simulink model "AdaptiveSIL"  (R2024a)
settings: Solver=VariableStepAuto  StartTime=0.0  StopTime=10  RelTol=1e-3
values from neighbouring files (symbols this model uses):
  am = 1/(Rlnom*C)    (= 53.1914893617)    [params.m]
  bm = 1    [params.m]
  C = 470e-6    (= 0.00047)    [params.m]
  k1 = 5000000    [params.m]
  k2 = 400000    [params.m]
  k3 = 700000    [params.m]
  kappa = 320    [params.m]
  L = 0.5e-3    (= 0.0005)    [params.m]
  omega = 100*pi    (= 314.159265359)    [params.m]
  Qas = bm    (= 1)    [params.m]
  R = 0.1    [params.m]
  Rlnom = 40    [params.m]
  Thetaas = 0    [params.m]
  vod = 200    [params.m]
libraries: eeTransforms x2, pspsim x1, spsSVPWMGenerator2LevelLib x1, spspowerguiLib x1
settings Model: Creator=CIO  LastModifiedBy=rodol
settings DebuggingCC: UnconnectedInputMsg=warning  UnconnectedOutputMsg=warning  UnconnectedLineMsg=warning
settings ModelReferenceCC: EnableRefExpFcnMdlSchedulingChecks=on
settings RTWCC: GPUComputeCapability=3.5  DLArmComputeVersion=19.05

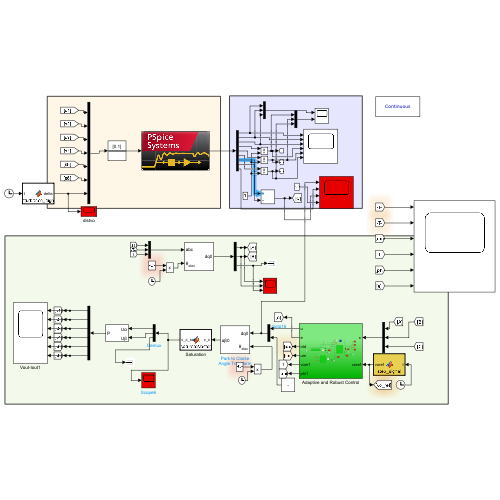
[thumbnail: Simulink's stored preview of the top-level diagram]
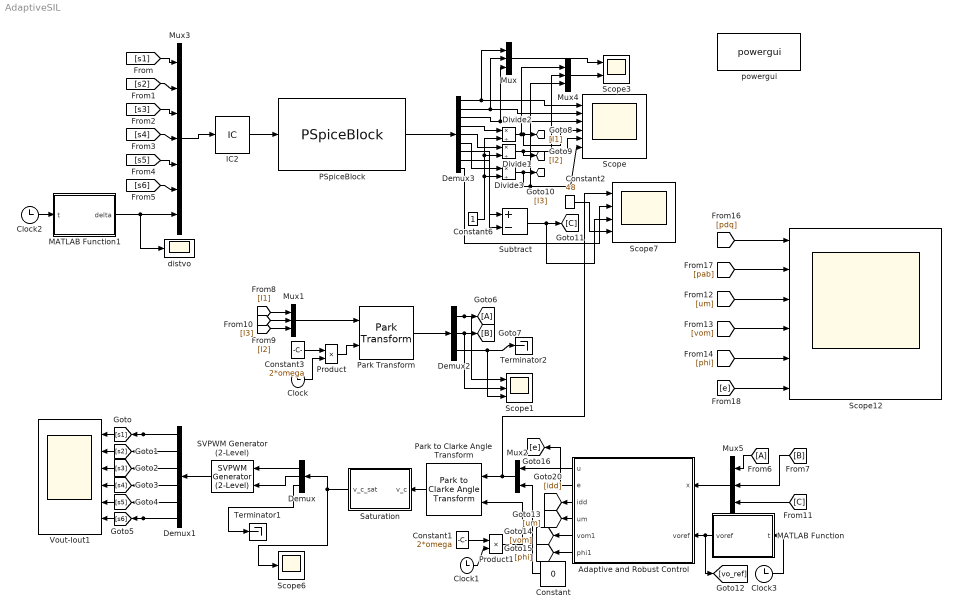
== system AdaptiveSIL ==
  Adaptive and Robust Control : Subsystem
  Clock{,1..3} (4 alike) : Clock
  Constant : Constant  Value=0
  Constant1 : Constant  Value=2*omega
  Constant2 : Constant  Value=48
  Constant3 : Constant  Value=2*omega
  Constant6 : Constant
  Demux : Demux  Outputs=3
  Demux1 : Demux  Outputs=6
  Demux2 : Demux  Outputs=3
  Demux3 : Demux  Outputs=9
  Divide1 : Product  Inputs=*/
  Divide2 : Product  Inputs=*/
  Divide3 : Product  Inputs=*/
  From6 : From
  Goto6 : Goto
  IC2 : InitialCondition  Value=0.1
  MATLAB Function : MATLAB Function  TreatAsAtomicUnit=on
  MATLAB Function1 : MATLAB Function  TreatAsAtomicUnit=on
  Mux{,1,4..5} (4 alike) : Mux  Inputs=3
  Mux2 : Mux  Inputs=2
  Mux3 : Mux  Inputs=7
  PSpiceBlock : pspsim/PSpiceBlock  SFunctionModules=''
      settings: SourceProductName=PSpice Block
  Park Transform : eeTransforms/Park Transform  AxisAlignment=D-axis  PowerInvariant=off
  Park to Clarke Angle Transform : eeTransforms/Park to Clarke Angle Transform  AxisAlignment=D-axis
  Product : Product
  Product1 : Product
  SVPWM Generator (2-Level) : spsSVPWMGenerator2LevelLib/SVPWM Generator (2-Level)  InputType=alpha-beta components  SwitchingPattern=Pattern #1  Fc=10000  ParUref=[0.8 -30 50]  Ts=0
  Saturation : MATLAB Function  TreatAsAtomicUnit=on
  Scope : Scope  NumInputPorts=6
  Scope1 : Scope  NumInputPorts=3
  Scope12 : Scope  NumInputPorts=6
  Scope3 : Scope  NumInputPorts=2
  Scope6 : Scope
  Scope7 : Scope  NumInputPorts=4
  Subtract : Sum  Inputs=+-
  Terminator1 : Terminator
  Terminator2 : Terminator
  Vout-Iout1 : Scope  NumInputPorts=6
  distvo : Scope
  powergui : spspowerguiLib/powergui  Priority=1  SimulationMode=Continuous  SampleTime=2e-6  frequency=60  Iterations=50  frequencyindice=60  Pbase=100e6  ErrMax=1e-4  UnitsV=kV  UnitsW=MW  buscounter=0  FunctionMessages=off  echomessages=off  EnableUseOfTLC=off  CurrentSourceSwitches=off  DisableSnubberDevices=off  DisableRonSwitches=off  DisableVfSwitches=off  DisplayEquations=off  AutomaticDiscreteSolvers=off  SolverType=Tustin/Backward Euler (TBE)  Interpol=off  ExternalGateDelay=off  methode=off  Ts=0  x0status=blocks  SPID=off  SwTol=0  HookPort=off  NonlinearTolerance=0  nMaxIteration=15  ContinueOnMaxIteration=off  RestoreLinks=warning  ResistiveCurrentMeasurement=off  Frange=[0:2:500]  Ylog=off  Xlog=on  ShowGrid=off  save=off  variable=ZData  structure=0  ZoomFFT=on  StartTime=0.0  cycles=1  DisplayStyle=1  fundamental=60  FreqAxis=off  MaxFrequency=1000  frequencyindicesteady=1  RmsSteady=1  display=off
  wires:
  Demux1/3 -> Vout-Iout1/3, [s3]
  [s1] -> Mux3/1
  [I1] -> Mux1/1
  Demux1/5 -> [s5], Vout-Iout1/5
  [s6] -> Mux3/6
  Demux/2 -> SVPWM Generator (2-Level)/2
  Demux/3 -> Terminator1/1
  [s4] -> Mux3/4
  Demux1/2 -> Vout-Iout1/2, [s2]
  Product1/1 -> Park to Clarke Angle Transform/2
  [s5] -> Mux3/5
  Park Transform/1 -> Demux2/1
  Mux2/1 -> Park to Clarke Angle Transform/1, Scope7/1
  Product/1 -> Park Transform/2
  Clock1/1 -> Product1/2
  [s3] -> Mux3/3
  Mux1/1 -> Park Transform/1
  Demux1/6 -> [s6], Vout-Iout1/6
  Demux2/2 -> Scope1/2, [B]
  Demux2/3 -> Scope1/3, Terminator2/1
  Demux/1 -> SVPWM Generator (2-Level)/1
  [I2] -> Mux1/2
  Demux1/1 -> Vout-Iout1/1, [s1]
  Clock/1 -> Product/2
  Demux2/1 -> Scope1/1, Goto6/1
  Mux3/1 -> IC2/1
  Constant1/1 -> Product1/1
  Demux1/4 -> Vout-Iout1/4, [s4]
  Constant3/1 -> Product/1
  [I3] -> Mux1/3
  [s2] -> Mux3/2
  IC2/1 -> PSpiceBlock/1
  PSpiceBlock/1 -> Demux3/1
  Demux3/1 -> Mux/1, Scope/1
  Demux3/2 -> Mux/2, Scope/2
  Demux3/3 -> Scope/3, Mux/3
  Demux3/7 -> Subtract/1
  Demux3/8 -> Subtract/2
  Demux3/4 -> Divide2/1
  Demux3/5 -> Divide1/1
  Demux3/6 -> Divide3/1
  Constant6/1 -> Divide3/2, Divide1/2, Divide2/2
  Divide2/1 -> Mux4/1, Scope/4, [I1]
  Divide1/1 -> [I2], Mux4/2, Scope/5
  Divide3/1 -> Scope/6, Mux4/3, [I3]
  Subtract/1 -> Scope7/3, [C]
  Constant2/1 -> Scope7/4
  Demux3/9 -> Scope7/2
  Mux4/1 -> Scope3/2
  Mux/1 -> Scope3/1
  MATLAB Function/1(voref) -> [vo_ref], Adaptive and Robust Control/2(voref)
  Clock3/1 -> MATLAB Function/1(t)
  Mux5/1 -> Adaptive and Robust Control/1(x)
  From6/1 -> Mux5/1
  [B] -> Mux5/2
  [C] -> Mux5/3
  Constant/1 -> Mux2/2
  Adaptive and Robust Control/1(u) -> Mux2/1
  SVPWM Generator (2-Level)/1 -> Demux1/1
  Park to Clarke Angle Transform/1 -> Saturation/1(v_c)
  Saturation/1(v_c_sat) -> Demux/1, Scope6/1
  Clock2/1 -> MATLAB Function1/1(t)
  MATLAB Function1/1(delta) -> distvo/1, Mux3/7
  [pdq] -> Scope12/1
  [pab] -> Scope12/2
  [um] -> Scope12/3
  [phi] -> Scope12/5
  [vom] -> Scope12/4
  [e] -> Scope12/6
  Adaptive and Robust Control/3(idd) -> [idd]
  Adaptive and Robust Control/4(um) -> [um]
  Adaptive and Robust Control/6(phi1) -> [phi]
  Adaptive and Robust Control/5(vom1) -> [vom]
  Adaptive and Robust Control/2(e) -> [e]

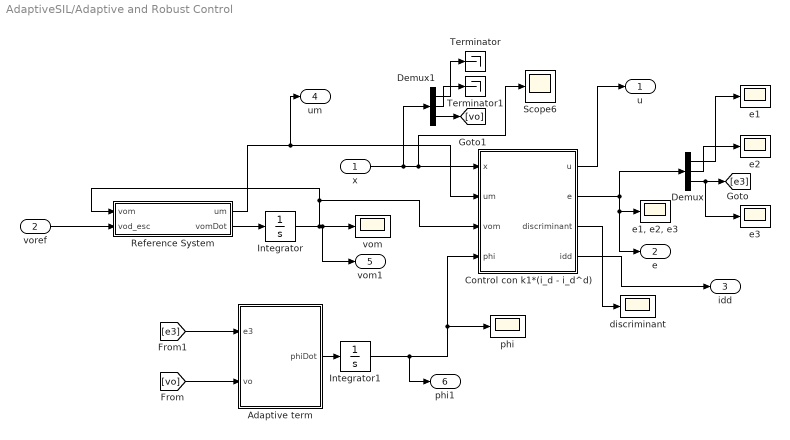
== system AdaptiveSIL/Adaptive and Robust Control ==
  x : Inport
  voref : Inport  Port=2
  " e1" : Scope
  " e2" : Scope
  " e3" : Scope
  Adaptive term : MATLAB Function  TreatAsAtomicUnit=on
  Control con k1*(i_d - i_d^d) : MATLAB Function  TreatAsAtomicUnit=on
  Demux : Demux  Outputs=3
  Demux1 : Demux  Outputs=3
  Integrator : Integrator
  Integrator1 : Integrator
  Reference System : MATLAB Function  TreatAsAtomicUnit=on
  Scope6 : Scope
  Terminator : Terminator
  Terminator1 : Terminator
  discriminant : Scope
  "e1, e2, e3" : Scope
  phi : Scope
  vom : Scope
  u : Outport
  e : Outport  Port=2
  idd : Outport  Port=3
  um : Outport  Port=4
  vom1 : Outport  Port=5
  phi1 : Outport  Port=6
  wires:
  x/1 -> Demux1/1, Scope6/1, Control con k1*(i_d - i_d^d)/1(x)
  Control con k1*(i_d - i_d^d)/3(discriminant) -> discriminant/1
  Control con k1*(i_d - i_d^d)/2(e) -> e/1, "e1, e2, e3"/1, Demux/1
  Control con k1*(i_d - i_d^d)/1(u) -> u/1
  Reference System/2(vomDot) -> Integrator/1
  Integrator/1 -> vom1/1, vom/1, Reference System/1(vom), Control con k1*(i_d - i_d^d)/3(vom)
  Adaptive term/1(phiDot) -> Integrator1/1
  Reference System/1(um) -> um/1, Control con k1*(i_d - i_d^d)/2(um)
  Integrator1/1 -> phi1/1, phi/1, Control con k1*(i_d - i_d^d)/4(phi)
  Demux/3 -> " e3"/1, [e3]
  Demux1/3 -> [vo]
  [e3] -> Adaptive term/1(e3)
  [vo] -> Adaptive term/2(vo)
  Demux1/1 -> Terminator/1
  Demux1/2 -> Terminator1/1
  voref/1 -> Reference System/2(vod_esc)
  Demux/1 -> " e1"/1
  Demux/2 -> " e2"/1
  Control con k1*(i_d - i_d^d)/4(idd) -> idd/1

== matlab function AdaptiveSIL/Adaptive and Robust Control/Reference System ==
  data: um output; vom input; vomDot output; am parameter; bm parameter; kappa parameter; vod_esc input
function [um, vomDot] = ref(vom, am, bm, kappa, vod_esc)

% Control
um = (1/bm)*( am*vom - kappa*(vom - vod_esc) );

% System
vomDot = - am*vom + bm*um ;

== matlab function AdaptiveSIL/MATLAB Function1 ==
  settings: updateMethod=DISCRETE
  data: t input; delta output
function delta = disturbance_signal(t)
% Disturbance and load variation signal approximation

% Componente suave (función senoidal con pendiente)
delta_base = 30*sin(0.7*t) + 5*t -20;

% Componente de ruido o pequeñas variaciones escalonadas:
% (simulando pequeños saltos pseudo-aleatorios)
rng(1); % Para reproducibilidad
persistent steps times
if isempty(steps)
    times = 0:0.09:10;
    steps = 0.1*(randn(size(times))); % valores aleatorios pequeños
end

% Interpolación para el valor de la señal escalonada en el tiempo t
noise_val = interp1(times, steps, t, 'previous', 0);

% Combinación final
delta = delta_base + noise_val;

end

== matlab function AdaptiveSIL/Adaptive and Robust Control/Control con k1*(i_d - i_d^d) ==
  data: x input; um input; vom input; phi input; u output; k1 parameter; k2 parameter; k3 parameter; vod parameter; R parameter; L parameter; C parameter; Rlnom parameter; omega parameter; E parameter; e output; discriminant output; Thetaas parameter; Qas parameter; idd output
function [u, e, discriminant,idd] = ctrl(x, um, vom, phi, k1, k2, k3, vod, R, L, C, Rlnom, omega, E, Thetaas, Qas)

id = x(1,1);
iq = x(2,1); 
vo = x(3,1);

% Errors e2, e3
e2 = iq;        e3 = vo - vom;
Theta = phi + Thetaas;

% Controls [Adaptive terms]
pq = ( (2*L)/(e3 + vom) )*( - (R/L)*iq - omega*id + k2*e2 ) ; % k2*e2 , k2*sqrt(abs(e2))*sign(e2)
v2 = Theta*vo + Qas*um  - (3/(4*C))*(iq*pq) - k3*e3 ;  % k3*e3 , k3*sqrt(abs(e3))*sign(e3)
%
%pq = ( 2*L/vo )*( - (R/L)*iq - omega*id + k2*sqrt(abs(e2))*sign(e2) ) ; % k2*e2 , k2*sqrt(abs(e2))*sign(e2)
%v2 = - (3/(4*C))*(iq*pq) + (1/(Rl*C))*vo - k3*sqrt(abs(e3))*sign(e3) ;  % k3*e3 , k3*sqrt(abs(e3))*sign(e3)

% Combinando las sigs. eqs (23) [version no adaptiva]
% pd = ((2*L)/(vo)) * ( - (R/L)*id + omega*iq + (E/L) + k1*(id - idd) ) ;
% idd = (4*C*v2)/(3*pd) ; 
% obtenemos:

a = k1;
b = (R/L) * id - omega * iq - (E/L) - k1 * id;
c = (2 * C * v2 * vo) / (3 * L);
discriminant = b^2 - 4 * a * c; %no debe ser cero

idd = ( -b + sqrt(b^2 - 4 * a * c) ) / (2 * a); %id deseada dinamica

pd = (4 * C * v2) / (3 * idd); %sale de (23)------------------> CONTROL REAL

% Error e1
e1 = id - idd;


% Salidas
u = [pd;
     pq];

e = [e1;
     e2;
     e3];

== matlab function AdaptiveSIL/Adaptive and Robust Control/Adaptive term ==
  data: e3 input; phiDot output; vo input; lambda parameter
function phiDot = fcn(e3, vo, lambda)


phiDot = - lambda*e3*vo;

== matlab function AdaptiveSIL/MATLAB Function ==
  data: t input; voref output; vod parameter
function voref = step_signal(t, vod)
% Generates a step signal increasing from 160 to 220 in steps of 20
% over a simulation time of 0 to 10 seconds.

    % Define step times and corresponding values
    %step_times = [0, 3.3, 6.6, 10]; % Change points
    %step_values = [vod-40, vod-20, vod, vod]; % Corresponding values
    step_times = [0, 2, 4, 6, 8]; % Change points
    %step_values = [vod-40, vod-20, vod, vod+20, vod+40]; % Corresponding values
    step_values = [vod, vod+20, vod+40, vod+80, vod+40]; % Corresponding values
    
    % Initialize output
    voref = step_values(1);
    
    % Apply step changes
    for i = 2:length(step_times)
        if t >= step_times(i)
            voref = step_values(i);
        end
    end
end

== matlab function AdaptiveSIL/Saturation ==
  data: v_c input; v_c_sat output
function v_c_sat = saturateVector(v_c)
%#codegen

% Separar componentes del vector
p_alpha = v_c(1);
p_beta = v_c(2);

% Calcular la magnitud
v_mag = sqrt(p_alpha^2 + p_beta^2);

% Máxima magnitud permitida
V_max = 0.866;

% Escalado si excede el límite
if v_mag <= V_max
    v_c_sat = v_c;
else
    scale = V_max / v_mag;
    v_c_sat = v_c * scale;
end
